simulink model "hw1_satellite"  (R2017a)
settings: Solver=ode45  StartTime=0.0  StopTime=5  RelTol=1e-3  EnableMultiTasking=on
InitFcn:
  | a = 5;
  | U = 1;
libraries: simulink x1
settings Model: Creator=edward  LastModifiedBy=edward
settings DataIOCC: LimitDataPoints=on  SaveFormat=Array
settings OptimizationCC: LifeSpan=inf
settings DebuggingCC: UnderspecifiedInitializationDetection=Classic  MergeDetectMultiDrivingBlocksExec=none  MaxConsecutiveZCsMsg=none  SolverPrmCheckMsg=warning  SFUnexpectedBacktrackingDiag=warning  SFNoUnconditionalDefaultTransitionDiag=warning  SFExecutionAtInitializationDiag=none
settings HardwareCC: ProdBitPerPointer=32  ProdBitPerSizeT=32  ProdBitPerPtrDiffT=32  ProdLargestAtomicFloat=None  ProdIntDivRoundTo=Undefined  ProdEndianess=Unspecified  ProdWordSize=32  ProdHWDeviceType=32-bit Generic
settings ModelReferenceCC: PropagateSignalLabelsOutOfModel=off
settings GRTTargetCC: TargetLangStandard=C89/C90 (ANSI)  GeneratePreprocessorConditionals=Disable all
settings ConfigComp: CovMetricSettings=dw  CovHtmlReporting=on  CovSaveCumulativeToWorkspaceVar=on  CovSaveSingleToWorkspaceVar=on  CovExternalEMLEnable=off

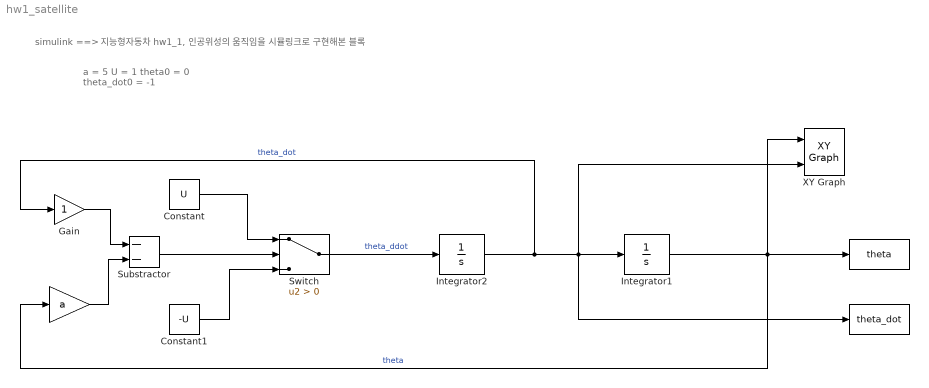
== system hw1_satellite ==
  note: a = 5
      | U = 1
      | theta0 = 0
      | theta_dot0 = -1
  note: simulink ==> 지능형자동차 hw1_1, 인공위성의 움직임을 시뮬링크로 구현해본 블록
  " " : Gain  Gain=a
  "  " : ToWorkspace  VariableName=theta  SaveFormat=Timeseries  SampleTime=-1
  "   " : ToWorkspace  VariableName=theta_dot  SaveFormat=Timeseries  SampleTime=-1
  Constant : Constant  Value=U
  Constant1 : Constant  Value=-U
  Gain : Gain
  Integrator1 : Integrator
  Integrator2 : Integrator  InitialCondition=-1
  "Substractor " : Sum  Inputs=--
  Switch : Switch  Criteria=u2 > Threshold
  XY Graph : simulink/Sinks/XY Graph  xmin=-1  xmax=1  ymin=-1  ymax=1  st=-1
  wires:
  Integrator2/1 -> Gain/1, "   "/1, XY Graph/2, Integrator1/1  "theta_dot"
  Integrator1/1 -> " "/1, "  "/1, XY Graph/1  "theta"
  Switch/1 -> Integrator2/1  "theta_ddot"
  " "/1 -> "Substractor "/2
  Constant/1 -> Switch/1
  Constant1/1 -> Switch/3
  Gain/1 -> "Substractor "/1
  "Substractor "/1 -> Switch/2
